simulink model "untitled"  (R2014a)
settings: Solver=ode45  StartTime=0.0  StopTime=10.0  RelTol=1e-3
libraries: powerlib x13
settings Model: Creator=503  LastModifiedBy=503

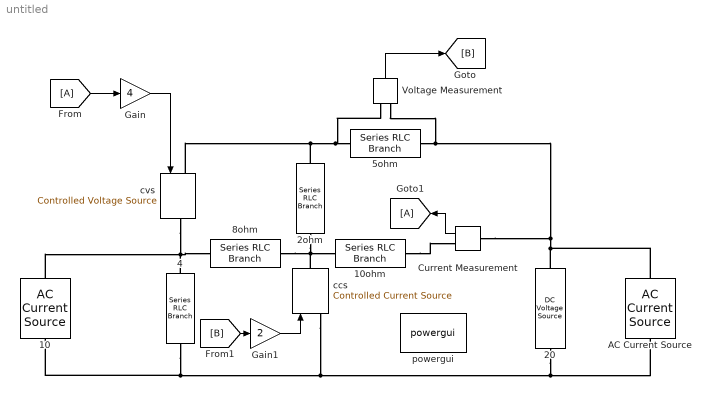
== system untitled ==
  10 : powerlib/Electrical Sources/AC Current Source  Amplitude=10  Phase=90  Frequency=0  SampleTime=0  Measurements=None
  "10ohm " : powerlib/Elements/Series RLC Branch  LConnTagsString=__new0  RConnTagsString=__new0  BranchType=R  Resistance=10  Inductance=1e-3  SetiL0=off  InitialCurrent=0  Capacitance=1e-6  Setx0=off  InitialVoltage=0  Measurements=None
  20 : powerlib/Electrical Sources/DC Voltage Source  Amplitude=100  Measurements=None
  2ohm : powerlib/Elements/Series RLC Branch  LConnTagsString=__new0  RConnTagsString=__new0  BranchType=R  Resistance=2  Inductance=1e-3  SetiL0=off  InitialCurrent=0  Capacitance=1e-6  Setx0=off  InitialVoltage=0  Measurements=None
  4 : powerlib/Elements/Series RLC Branch  LConnTagsString=__new0  RConnTagsString=__new0  BranchType=R  Resistance=4  Inductance=1e-3  SetiL0=off  InitialCurrent=0  Capacitance=1e-6  Setx0=off  InitialVoltage=0  Measurements=None
  5ohm : powerlib/Elements/Series RLC Branch  LConnTagsString=__new0  RConnTagsString=__new0  BranchType=R  Resistance=5  Inductance=1e-3  SetiL0=off  InitialCurrent=0  Capacitance=1e-6  Setx0=off  InitialVoltage=0  Measurements=None
  8ohm : powerlib/Elements/Series RLC Branch  LConnTagsString=__new0  RConnTagsString=__new0  BranchType=R  Resistance=8  Inductance=1e-3  SetiL0=off  InitialCurrent=0  Capacitance=1e-6  Setx0=off  InitialVoltage=0  Measurements=None
  AC Current Source : powerlib/Electrical Sources/AC Current Source  Amplitude=6  Phase=90  Frequency=0  SampleTime=0  Measurements=None
  Current Measurement : powerlib/Measurements/Current Measurement  PhasorSimulation=off  OutputType=Complex  PSBequivalent=0
  Gain : Gain  Gain=4
  Gain1 : Gain  Gain=2
  Voltage Measurement : powerlib/Measurements/Voltage Measurement  PhasorSimulation=off  OutputType=Complex  PSBequivalent=0
  ccs : powerlib/Electrical Sources/Controlled Current Source  Initialize=on  Source_Type=AC  Amplitude=0  Phase=0  Frequency=0  Measurements=None
  cvs : powerlib/Electrical Sources/Controlled Voltage Source  Initialize=on  Source_Type=AC  Amplitude=0  Phase=0  Frequency=0  Measurements=None
  powergui : powerlib/powergui  Priority=1  SimulationMode=Continuous  SolverType=Tustin  SampleTime=50e-6  frequency=60  SPID=off  DisableSnubberDevices=off  DisableRonSwitches=off  DisableVfSwitches=off  SwTol=0  Interpol=off  DisplayEquations=off  Ts=0  methode=off  frequencyindice=0  Pbase=100e6  ErrMax=1e-4  Iterations=50  UnitsV=kV  UnitsW=MW  FunctionMessages=off  echomessages=off  HookPort=off  EnableUseOfTLC=off  x0status=blocks  RestoreLinks=warning  ResistiveCurrentMeasurement=off  Frange=[0:2:500]  Ylog=off  Xlog=on  ShowGrid=off  save=off  variable=ZData  structure=0  ZoomFFT=off  StartTime=0.0  cycles=1  DisplayStyle=1  fundamental=60  FreqAxis=off  MaxFrequency=1000  frequencyindicesteady=1  RmsSteady=1  display=off
  wires:
  [A] -> Gain/1
  [B] -> Gain1/1
  Gain1/1 -> ccs/1
  Gain/1 -> cvs/1
  Voltage Measurement/1 -> [B]
  Current Measurement/1 -> [A]
  connections:
  8ohm/LConn1 -- ccs/RConn1 -- 2ohm/RConn1 -- "10ohm "/LConn1
  2ohm/LConn1 -- Voltage Measurement/LConn1 -- 5ohm/LConn1 -- cvs/LConn1
  5ohm/RConn1 -- Voltage Measurement/LConn2 -- 20/RConn1 -- AC Current Source/RConn1 -- Current Measurement/LConn1
  4/RConn1 -- ccs/LConn1 -- 20/LConn1 -- AC Current Source/LConn1 -- 10/LConn1
  4/LConn1 -- 10/RConn1 -- cvs/RConn1 -- 8ohm/RConn1
  "10ohm "/RConn1 -- Current Measurement/RConn1
